simulink model "CubaModelPID"  (R2016a)
settings: Solver=FixedStepAuto  StartTime=0.0  StopTime=3  FixedStep=0.001  RelTol=1e-3
values from neighbouring files (symbols this model uses):
  C_b = 2.1e-3    (= 0.0021)    [configurePID.m]
  C_w = 2.1268e-5    (= 2.1268e-05)    [configurePID.m]
  g = 9.81    [configurePID.m]
  l = 0.08455    [configurePID.m]
  l_b = 0.0751442    [configurePID.m]
  m_b = 0.294    [configurePID.m]
  m_w = 0.1298    [configurePID.m]
  O_G_A = O_b_A + m_w * l^2    (= 0.0042279015845)    [configurePID.m]
  O_w_B = 0.088e-3    (= 8.8e-05)    [configurePID.m]
  phi_b0 = degtorad(1)    [configurePID.m]
  phi_b__d0 = degtorad(0)    [configurePID.m]
  phi_w0 = degtorad(0)    [configurePID.m]
  phi_w__d0 = degtorad(0)    [configurePID.m]
  T_M_e = 5.5e-4    (= 0.00055)    [configurePID.m]
  T_M_m = 12.4e-3    (= 0.0124)    [configurePID.m]
undefined symbols (not defined in the file or in its folder): degtorad
settings Model: Creator=michael  LastModifiedBy=ich

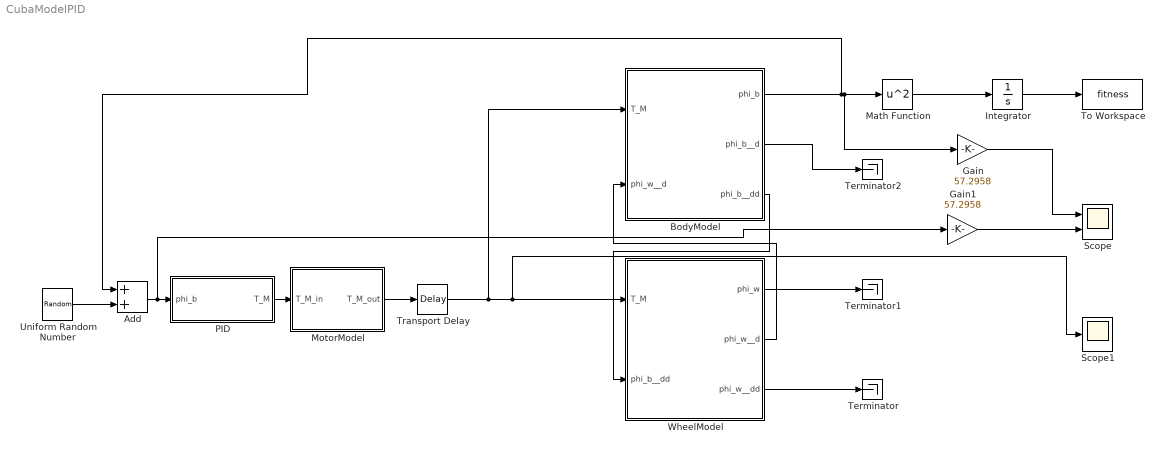
== system CubaModelPID ==
  Add : Sum
  BodyModel : Subsystem
  Gain : Gain  Gain=57.2958
  Gain1 : Gain  Gain=57.2958
  Integrator : Integrator
  Math Function : Math  Operator=square  SaturateOnIntegerOverflow=on
  "MotorModel " : Subsystem
  PID : Subsystem
  Scope : Scope  NumInputPorts=2
  Scope1 : Scope
  Terminator : Terminator
  Terminator1 : Terminator
  Terminator2 : Terminator
  To Workspace : ToWorkspace  VariableName=fitness  SampleTime=-1
      settings: MaxDataPoints=1
  Transport Delay : TransportDelay  DelayTime=0.01
  Uniform Random Number : UniformRandomNumber  Minimum=-(degtorad(0.2))  Maximum=degtorad(0.2)  SampleTime=0.001
  WheelModel : Subsystem
  wires:
  WheelModel/2(phi_w__d) -> BodyModel/2(phi_w__d)
  BodyModel/3(phi_b__dd) -> WheelModel/2(phi_b__dd)
  BodyModel/1(phi_b) -> Add/1, Gain/1, Math Function/1
  PID/1(T_M) -> "MotorModel "/1(T_M_in)
  Math Function/1 -> Integrator/1
  Integrator/1 -> To Workspace/1
  "MotorModel "/1(T_M_out) -> Transport Delay/1
  BodyModel/2(phi_b__d) -> Terminator2/1
  WheelModel/1(phi_w) -> Terminator1/1
  WheelModel/3(phi_w__dd) -> Terminator/1
  Add/1 -> Gain1/1, PID/1(phi_b)
  Uniform Random Number/1 -> Add/2
  Transport Delay/1 -> BodyModel/1(T_M), Scope1/1, WheelModel/1(T_M)
  Gain/1 -> Scope/1
  Gain1/1 -> Scope/2

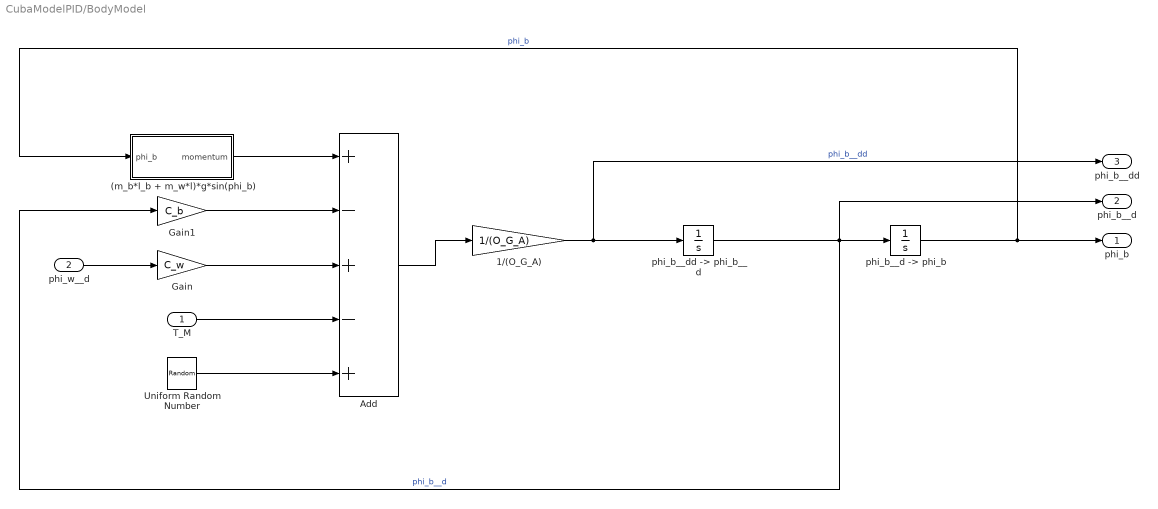
== system CubaModelPID/BodyModel ==
  T_M : Inport
  phi_w__d : Inport  Port=2
  (m_b*l_b + m_w*l)*g*sin(phi_b) : Subsystem
  1/(O_G_A) : Gain  Gain=1/(O_G_A)
  Add : Sum  Inputs=+-+-+
  Gain : Gain  Gain=C_w
  Gain1 : Gain  Gain=C_b
  Uniform Random Number : UniformRandomNumber  Minimum=-0.01  Maximum=0.01  SampleTime=0.001
  "phi_b__d -> phi_b" : Integrator  InitialCondition=phi_b0
  "phi_b__dd -> phi_b__d" : Integrator  InitialCondition=phi_b__d0
  phi_b : Outport
  phi_b__d : Outport  Port=2
  phi_b__dd : Outport  Port=3
  wires:
  T_M/1 -> Add/4
  Gain/1 -> Add/3
  Gain1/1 -> Add/2
  (m_b*l_b + m_w*l)*g*sin(phi_b)/1(momentum) -> Add/1
  phi_w__d/1 -> Gain/1
  Add/1 -> 1/(O_G_A)/1
  1/(O_G_A)/1 -> phi_b__dd/1, "phi_b__dd -> phi_b__d"/1  "phi_b__dd"
  "phi_b__dd -> phi_b__d"/1 -> Gain1/1, phi_b__d/1, "phi_b__d -> phi_b"/1  "phi_b__d"
  "phi_b__d -> phi_b"/1 -> phi_b/1, (m_b*l_b + m_w*l)*g*sin(phi_b)/1(phi_b)  "phi_b"
  Uniform Random Number/1 -> Add/5

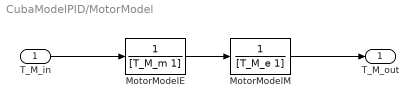
== system CubaModelPID/MotorModel  ==
  T_M_in : Inport
  MotorModelE : TransferFcn  Denominator=[T_M_m 1]
  MotorModelM : TransferFcn  Denominator=[T_M_e 1]
  T_M_out : Outport
  wires:
  MotorModelE/1 -> MotorModelM/1
  T_M_in/1 -> MotorModelE/1
  MotorModelM/1 -> T_M_out/1

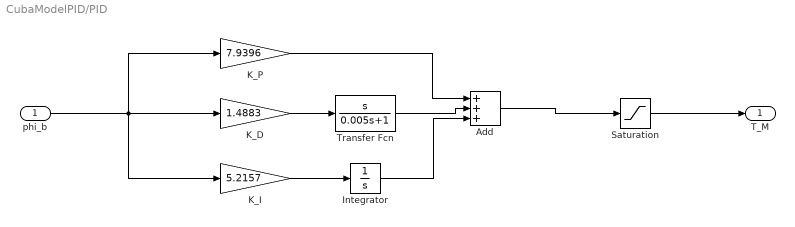
== system CubaModelPID/PID ==
  phi_b : Inport
  Add : Sum  Inputs=+++
  Integrator : Integrator
  K_D : Gain  Gain=1.4883
  K_I : Gain  Gain=5.2157
  K_P : Gain  Gain=7.9396
  Saturation : Saturate  UpperLimit=0.1  LowerLimit=-0.1
  Transfer Fcn : TransferFcn  Numerator=[1 0]  Denominator=[0.005 1]
  T_M : Outport
  wires:
  phi_b/1 -> K_I/1, K_P/1, K_D/1
  K_I/1 -> Integrator/1
  Add/1 -> Saturation/1
  K_D/1 -> Transfer Fcn/1
  K_P/1 -> Add/1
  Transfer Fcn/1 -> Add/2
  Saturation/1 -> T_M/1
  Integrator/1 -> Add/3

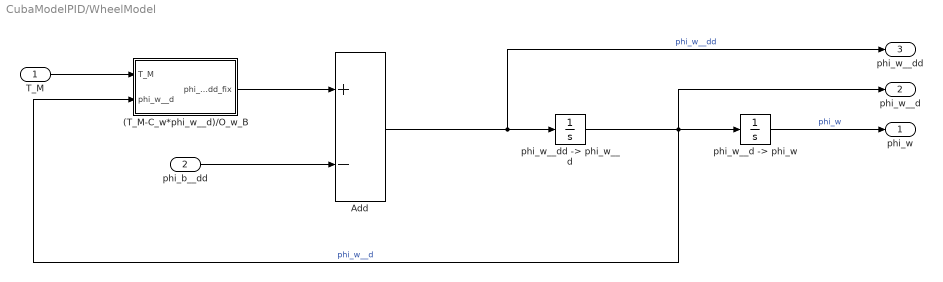
== system CubaModelPID/WheelModel ==
  T_M : Inport
  phi_b__dd : Inport  Port=2
  (T_M-C_w*phi_w__d)/O_w_B : Subsystem
  Add : Sum  Inputs=+-
  "phi_w__d -> phi_w" : Integrator  InitialCondition=phi_w0
  "phi_w__dd -> phi_w__d" : Integrator  InitialCondition=phi_w__d0
  phi_w : Outport
  phi_w__d : Outport  Port=2
  phi_w__dd : Outport  Port=3
  wires:
  phi_b__dd/1 -> Add/2
  Add/1 -> phi_w__dd/1, "phi_w__dd -> phi_w__d"/1  "phi_w__dd"
  "phi_w__dd -> phi_w__d"/1 -> phi_w__d/1, (T_M-C_w*phi_w__d)/O_w_B/2(phi_w__d), "phi_w__d -> phi_w"/1  "phi_w__d"
  (T_M-C_w*phi_w__d)/O_w_B/1(phi_w__dd_fix) -> Add/1
  T_M/1 -> (T_M-C_w*phi_w__d)/O_w_B/1(T_M)
  "phi_w__d -> phi_w"/1 -> phi_w/1  "phi_w"

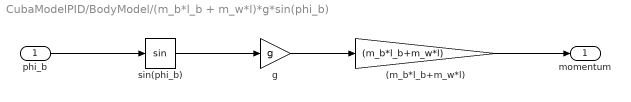
== system CubaModelPID/BodyModel/(m_b*l_b + m_w*l)*g*sin(phi_b) ==
  phi_b : Inport
  (m_b*l_b+m_w*l) : Gain  Gain=(m_b*l_b+m_w*l)
  g : Gain  Gain=g
  sin(phi_b) : Trigonometry
  momentum : Outport
  wires:
  sin(phi_b)/1 -> g/1
  phi_b/1 -> sin(phi_b)/1
  g/1 -> (m_b*l_b+m_w*l)/1
  (m_b*l_b+m_w*l)/1 -> momentum/1

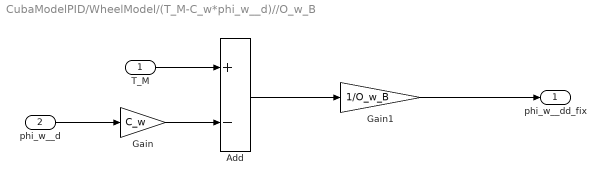
== system CubaModelPID/WheelModel/(T_M-C_w*phi_w__d)//O_w_B ==
  T_M : Inport
  phi_w__d : Inport  Port=2
  Add : Sum  Inputs=+-
  Gain : Gain  Gain=C_w
  Gain1 : Gain  Gain=1/O_w_B
  phi_w__dd_fix : Outport
  wires:
  T_M/1 -> Add/1
  phi_w__d/1 -> Gain/1
  Gain/1 -> Add/2
  Add/1 -> Gain1/1
  Gain1/1 -> phi_w__dd_fix/1
